simulink model "MPC_TRAJ"  (R2025b)
settings: Solver=VariableStepAuto  StartTime=0.0  StopTime=10  RelTol=1e-3
InitFcn:
  | clear; clc; close all;
  | 
  | % System parameters
  | m = 0.2;
  | M = 1;
  | g = 9.81;
  | bc = 0.1;
  | bp = 0.05;
  | l0 = 0.5;
  | theta0 = 0;
  | x0 = -0.5; % or -5
  | 
  | % NMPC horizons and constraints
  | Ts = 0.05;
  | prediction_horizon = 25;
  | control_horizon = 5;
  | 
  | theta_max = deg2rad(15);
  | theta_min = -theta_max;
  | l_max = 1.5; l_min = 0.1;
  | f_max = 50; f_min = -f_max;
  | l_ddot_max = 5; l_ddot_min = -l_ddot_max;
  | 
  | % NMPC object configuration
  | nx = 6; % States: [x, x_dot, theta, theta_dot, l, l_dot]
  | ny = 6; % Outputs
  | nu = 2; % Inputs: [F, l_ddot]
  | 
  | nlobj = nlmpc(nx, ny, nu);
  | nlobj.Model.StateFcn = "CraneStateFcn";
  | nlobj.Ts = Ts;
  | nlobj.PredictionHorizon = prediction_horizon;
  | nlobj.ControlHorizon = control_horizon;
  | 
  | % Set HARD state constraints
  | nlobj.States(3).Min = theta_min; nlobj.States(3).Max = theta_max;
  | nlobj.States(5).Min = l_min; nlobj.States(5).Max = l_max;
  | 
  | % Set MV hard constraints
  | nlobj.MV(1).Min = f_min; nlobj.MV(1).Max = f_max;
  | nlobj.MV(2).Min = l_ddot_min; nlobj.MV(2).Max = l_ddot_max;
  | 
  | % Distance-Invariant Tuning Weights
  | % OutputVariables: [x, x_dot, theta, theta_dot, l, l_dot]
  | % x weight reduced to allow tracking flexibility without constraint violation
  | nlobj.Weights.OutputVariables = [150, 20, 300, 20, 50, 10];
  | 
  | % ManipulatedVariables: [F, l_ddot]
  | nlobj.Weights.ManipulatedVariables = [1, 1];
  | 
  | % ManipulatedVariablesRate: [F_rate, l_ddot_rate]
  | % Heavily penalized to enforce smooth control actions, preventing hard constraint hits
  | nlobj.Weights.ManipulatedVariablesRate = [150, 150];
  | 
  | % Optimization solver settings
  | nlobj.Optimization.SolverOptions.Algorithm = 'sqp';
  | nlobj.Optimization.SolverOptions.MaxIterations = 200;
  | % Increase tolerance slightly to help the solver in tight constraint scenarios
  | nlobj.Optimization.SolverOptions.StepTolerance = 1e-4;
  | 
  | % Trajectory and feedforward parameters
  | v_max = 1.0;
  | a_max = 2.0;
  | traj_params = [x0, v_max, a_max, M, m, bc, l0];
model workspace (MAT data in the model file):
  Sig = Simulink.Signal
  Sig.Dimensions = -1
  Sig.DimensionsMode = 'auto'
  Sig.Complexity = 'auto'
  Sig.SampleTime = -1
  Sig.SamplingMode = 'auto'
  Sig.DataType = 'auto'
values from neighbouring files (symbols this model uses):
  L = x_target - x0    [TrajectoryGenerator.m]
  s = 10 * tau ^ 3 - 15 * tau ^ 4 + 6 * tau ^ 5    [TrajectoryGenerator.m]
undefined symbols (not defined in the file or in its folder): X, Y, Z
libraries: sm_lib x13, nesl_utility x7, mpclib x1
settings Model: Creator=JNemune  LastModifiedBy=JNemune

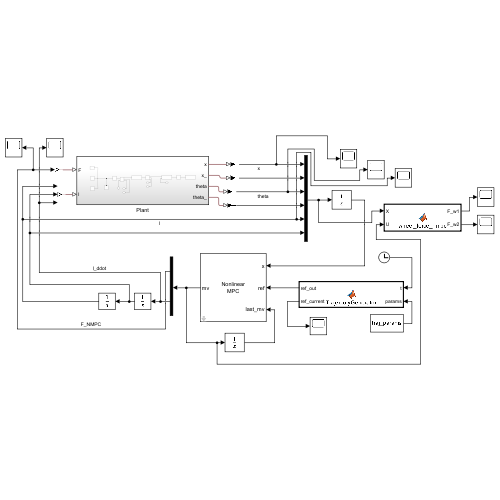
[thumbnail: Simulink's stored preview of the top-level diagram]
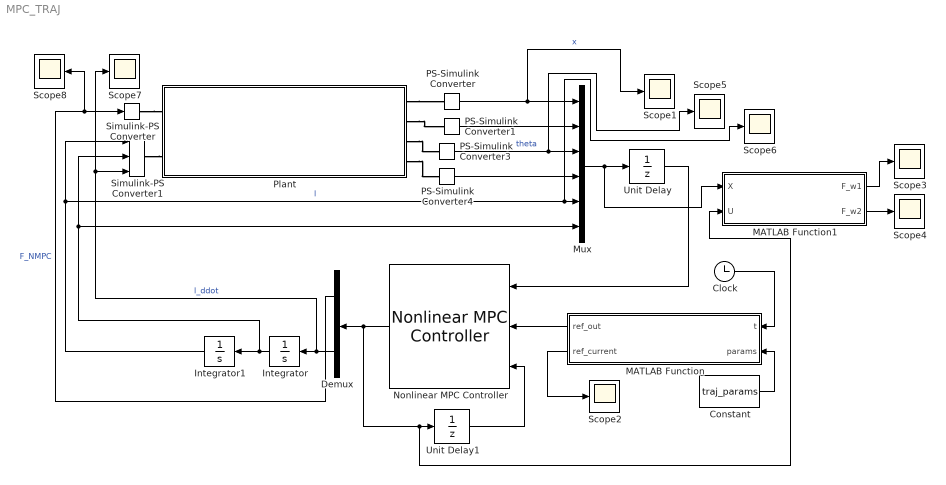
== system MPC_TRAJ ==
  Clock : Clock
  Constant : Constant  Value=traj_params
  Demux : Demux  Outputs=2
  Integrator : Integrator
  Integrator1 : Integrator  InitialCondition=l0
  MATLAB Function : MATLAB Function  TreatAsAtomicUnit=on
  MATLAB Function1 : MATLAB Function  TreatAsAtomicUnit=on
  Mux : Mux  Inputs=6
  Nonlinear MPC Controller : mpclib/Nonlinear MPC Controller  nlmpcobj=nlobj  UseObjectTs=on  UseMEX=off  md_enabled=off  mvtarget_enabled=off  param_enabled=off  cost_enabled=off  mvseq_enabled=off  stateseq_enabled=off  ovseq_enabled=off  slack_enabled=off  status_enabled=off  ov_min=off  ov_max=off  mv_min=off  mv_max=off  mvrate_min=off  mvrate_max=off  state_min=off  state_max=off  ov_weight=off  mv_weight=off  mvrate_weight=off  ecr_weight=off  nlp_initialize=off
  PS-Simulink Converter{,1,3..4} (4 alike) : nesl_utility/PS-Simulink Converter  PhysicalDomain=network_engine_domain  SubClassName=ps_output  LeftPortType=input  RightPortType=output  PseudoPeriodic=off  Frequencies=[]  VectorFormat=inherit  Unit=inherit  AffineConversion=off
  Plant : Subsystem
  Scope{1..8} (8 alike) : Scope
      Scope1 settings: Title=Plant Input (F, l_ddot)  ActiveDisplayYMinimum=-0.57069229240965214  ActiveDisplayYMaximum=0.1182567265577066
      Scope2 settings: ActiveDisplayYMinimum=-0.5625  ActiveDisplayYMaximum=0.062499999999999986  DataLoggingVariableName=ScopeData2
      Scope3 settings: Title=Plant Input (F, l_ddot)  ActiveDisplayYMinimum=5.8532583517724026  ActiveDisplayYMaximum=5.9075728848445683  DataLoggingVariableName=ScopeData3
      Scope4 settings: Title=Plant Input (F, l_ddot)  ActiveDisplayYMinimum=5.8611422440219316  ActiveDisplayYMaximum=5.9241092198238494  DataLoggingVariableName=ScopeData4
      Scope5 settings: Title=Plant Input (F, l_ddot)  ActiveDisplayYMinimum=-0.093511798344871486  ActiveDisplayYMaximum=0.060809549458767209
      Scope6 settings: Title=Plant Input (F, l_ddot)  ActiveDisplayYMinimum=0.49743738451947506  ActiveDisplayYMaximum=0.510974024582042  DataLoggingVariableName=ScopeData5
      Scope7 settings: Title=Plant Input (F, l_ddot)  ActiveDisplayYMinimum=-0.039593269711448255  ActiveDisplayYMaximum=0.049854556653327248  DataLoggingVariableName=ScopeData6
      Scope8 settings: Title=Plant Input (F, l_ddot)  ActiveDisplayYMinimum=-0.62140528534348749  ActiveDisplayYMaximum=0.7248047355020627  DataLoggingVariableName=ScopeData7
  Simulink-PS Converter : nesl_utility/Simulink-PS Converter  PhysicalDomain=network_engine_domain  SubClassName=ps_input  LeftPortType=input  RightPortType=output  PseudoPeriodic=off  Frequencies=[]  NoiseDistribution=none  NoiseParameters=[]  Unit=1  AffineConversion=off  FilteringAndDerivatives=provide  SimscapeFilterOrder=1  InputFilterTimeConstant=0.001  UdotUserProvided=0
  Simulink-PS Converter1 : nesl_utility/Simulink-PS Converter  PhysicalDomain=network_engine_domain  SubClassName=ps_input  LeftPortType=input  RightPortType=output  PseudoPeriodic=off  Frequencies=[]  NoiseDistribution=none  NoiseParameters=[]  Unit=1  AffineConversion=off  FilteringAndDerivatives=provide  SimscapeFilterOrder=1  InputFilterTimeConstant=0.001  UdotUserProvided=2
  Unit Delay : UnitDelay  InitialCondition=[0, 0, theta0, 0, l0, 0]  SampleTime=Ts  HasFrameUpgradeWarning=on
  Unit Delay1 : UnitDelay  InitialCondition=[0, 0]  SampleTime=Ts  HasFrameUpgradeWarning=on
  wires:
  PS-Simulink Converter1/1 -> Mux/2
  Integrator/1 -> Simulink-PS Converter1/2, Mux/6, Integrator1/1
  MATLAB Function/1(ref_out) -> Nonlinear MPC Controller/2
  Nonlinear MPC Controller/1 -> MATLAB Function1/2(U), Unit Delay1/1, Demux/1
  Integrator1/1 -> Simulink-PS Converter1/1, Scope6/1, Mux/5  "l"
  PS-Simulink Converter4/1 -> Mux/4
  Mux/1 -> MATLAB Function1/1(X), Unit Delay/1
  Unit Delay/1 -> Nonlinear MPC Controller/1
  Unit Delay1/1 -> Nonlinear MPC Controller/3
  PS-Simulink Converter3/1 -> Scope5/1, Mux/3  "theta"
  PS-Simulink Converter/1 -> Scope1/1, Mux/1  "x"
  Demux/2 -> Scope7/1, Simulink-PS Converter1/3, Integrator/1  "l_ddot"
  Demux/1 -> Scope8/1, Simulink-PS Converter/1  "F_NMPC"
  Clock/1 -> MATLAB Function/1(t)
  Constant/1 -> MATLAB Function/2(params)
  MATLAB Function/2(ref_current) -> Scope2/1
  MATLAB Function1/1(F_w1) -> Scope3/1
  MATLAB Function1/2(F_w2) -> Scope4/1
  connections:
  Plant/RConn2 -- PS-Simulink Converter1/LConn1
  Simulink-PS Converter1/RConn1 -- Plant/LConn2
  Simulink-PS Converter/RConn1 -- Plant/LConn1
  Plant/RConn3 -- PS-Simulink Converter3/LConn1
  Plant/RConn1 -- PS-Simulink Converter/LConn1
  Plant/RConn4 -- PS-Simulink Converter4/LConn1

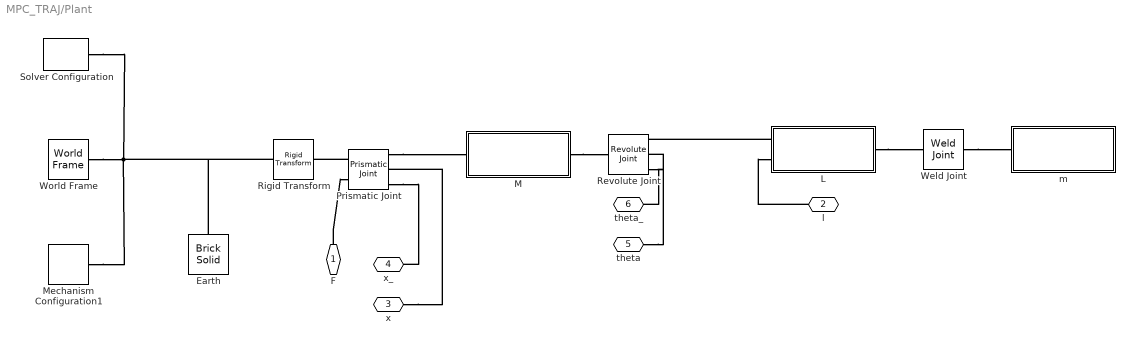
== system MPC_TRAJ/Plant ==
  Earth : sm_lib/Body Elements/Brick Solid  BrickDimensions=[1000 1 1]  BrickDimensionsUnits=mm  ExportEntireGeometry=off  InertiaType=CalculateFromGeometry  BasedOnType=Density  Density=1000  DensityUnits=kg/m^3  Mass=1  MassUnits=kg  CenterOfMass=[0 0 0]  CenterOfMassUnits=m  MomentsOfInertia=[1 1 1]  MomentsOfInertiaUnits=kg*m^2  ProductsOfInertia=[0 0 0]  ProductsOfInertiaUnits=kg*m^2  GraphicType=FromGeometry  MarkerShape=Sphere  MarkerSize=10  GraphicVisPropType=SimpleVisualProperties  GraphicDiffuseColor=[0.5 0.5 0.5]  GraphicOpacity=1.0  GraphicSpecularColor=[0.5 0.5 0.5 1.0]  GraphicAmbientColor=[0.15 0.15 0.15 1.0]  GraphicEmissiveColor=[0.0 0.0 0.0 1.0]  GraphicShininess=75  DoExposeReferenceFrame=on  SerializedFrames=<Frames/>
  L : Subsystem
  M : Subsystem
  Mechanism Configuration1 : sm_lib/Utilities/Mechanism Configuration  UniformGravity=Constant  GravityVector=[0 0 -g]  GravityVectorUnits=m/s^2  LinearizationDelta=0.001  JointModeTransitionNonlinearIterations=2
  Prismatic Joint : sm_lib/Joints/Prismatic Joint  JointMode=Normal  CompositeWrenchDir=FollowerOnBase  CompositeWrenchFrame=BaseFrame  SenseConstraintForce=off  SenseConstraintTorque=off  SenseTotalForce=off  SenseTotalTorque=off  PositionTargetSpecify=on  PositionTargetPriority=High  PositionTargetValue=x0  PositionTargetValueUnits=m  VelocityTargetSpecify=off  VelocityTargetPriority=High  VelocityTargetValue=0  VelocityTargetValueUnits=m/s  EquilibriumPosition=0  EquilibriumPositionUnits=m  SpringStiffness=0  SpringStiffnessUnits=N/m  DampingCoefficient=bc  DampingCoefficientUnits=N/(m/s)  LowerLimitSpecify=off  LowerLimitBound=-1  LowerLimitBoundUnits=m  LowerLimitStiffness=1e6  LowerLimitStiffnessUnits=N/m  LowerLimitDamping=1e3  LowerLimitDampingUnits=N/(m/s)  LowerLimitTransitionRegionWidth=1e-4  LowerLimitTransitionRegionWidthUnits=m  UpperLimitSpecify=off  UpperLimitBound=1  UpperLimitBoundUnits=m  UpperLimitStiffness=1e6  UpperLimitStiffnessUnits=N/m  UpperLimitDamping=1e3  UpperLimitDampingUnits=N/(m/s)  UpperLimitTransitionRegionWidth=1e-4  UpperLimitTransitionRegionWidthUnits=m  TorqueActuationMode=InputTorque  MotionActuationMode=ComputedMotion  SensePosition=on  SenseVelocity=on  SenseAcceleration=off  SenseTorqueForce=off  SenseLowerLimitTorqueForce=off  SenseUpperLimitTorqueForce=off
  Revolute Joint : sm_lib/Joints/Revolute Joint  JointMode=Normal  CompositeWrenchDir=FollowerOnBase  CompositeWrenchFrame=BaseFrame  SenseConstraintForce=off  SenseConstraintTorque=off  SenseTotalForce=off  SenseTotalTorque=off  PositionTargetSpecify=on  PositionTargetPriority=High  PositionTargetValue=theta0  PositionTargetValueUnits=rad  VelocityTargetSpecify=off  VelocityTargetPriority=High  VelocityTargetValue=0  VelocityTargetValueUnits=deg/s  EquilibriumPosition=0  EquilibriumPositionUnits=deg  SpringStiffness=0  SpringStiffnessUnits=N*m/deg  DampingCoefficient=bp  DampingCoefficientUnits=N*m*s/rad  LowerLimitSpecify=off  LowerLimitBound=-90  LowerLimitBoundUnits=deg  LowerLimitStiffness=1e4  LowerLimitStiffnessUnits=N*m/deg  LowerLimitDamping=10  LowerLimitDampingUnits=N*m/(deg/s)  LowerLimitTransitionRegionWidth=0.1  LowerLimitTransitionRegionWidthUnits=deg  UpperLimitSpecify=off  UpperLimitBound=90  UpperLimitBoundUnits=deg  UpperLimitStiffness=1e4  UpperLimitStiffnessUnits=N*m/deg  UpperLimitDamping=10  UpperLimitDampingUnits=N*m/(deg/s)  UpperLimitTransitionRegionWidth=0.1  UpperLimitTransitionRegionWidthUnits=deg  TorqueActuationMode=NoTorque  MotionActuationMode=ComputedMotion  SensePosition=on  SenseVelocity=on  SenseAcceleration=off  SenseTorqueForce=off  SenseLowerLimitTorqueForce=off  SenseUpperLimitTorqueForce=off
  Rigid Transform : sm_lib/Frames and Transforms/Rigid Transform  RotationMethod=StandardAxis  FollAlignAxisA=+X  BaseAlignAxisA=+Y  FollAlignAxisB=+Y  BaseAlignAxisB=+Z  RotationStandardAxis=+Y  RotationAngle=90  RotationAngleUnits=deg  RotationArbitraryAxis=[0 0 1]  RotationSequenceAxes=FollowerAxes  RotationSequence=XYX  RotationSequenceAngles=[0 0 0]  RotationSequenceAnglesUnits=deg  RotationMatrix=[1 0 0; 0 1 0; 0 0 1]  Quaternion=[1 0 0 0]  TranslationMethod=None  TranslationCartesianOffset=[x0 0 0]  TranslationCartesianOffsetUnits=m  TranslationStandardAxis=+Z  TranslationStandardOffset=0  TranslationStandardOffsetUnits=m  TranslationROffset=0  TranslationROffsetUnits=m  TranslationThetaOffset=0  TranslationThetaOffsetUnits=deg  TranslationZOffset=0  TranslationZOffsetUnits=m
  Solver Configuration : nesl_utility/Solver Configuration  PhysicalDomain=network_engine_domain  SubClassName=solver  LeftPortType=input  RightPortType=generic  Tones=[]  Harmonics=[]  SimulateNoise=off  Profile=off  UseLocalSampling=off  EnableSwitchedLinearOptims=on  FrequencyDomain=off  UseCCode=off  RelTol=0.001  AbsTol=0.001  MinStep=1e-09  ToWorkspace=off  RevertToSquareIcSolve=off  NumHomotopyIterations=100  PhasorMode=off  PhasorModeNumHarmonics=1  ConsistencySolver=NEWTON_XTOL_AFTER_FTOL  IndexReductionMethod=DerivativeReplacement  DoDC=off  ResidualTolerance=1e-09  ConsistencyTolSource=GLOBAL  ConsistencyAbsTol=0.001  ConsistencyRelTol=0.001  ConsistencyTolFactor=0.001  UseLocalSolver=off  LocalSolverChoice=NE_BACKWARD_EULER_ADVANCER  ResolveIndetEquations=on  FunctionEvalNumThread=1  LocalSolverSampleTime=0.001  DoFixedCost=off  MaxNonlinIter=3  MaxModeIter=2  ComputeImpulses=off  ImpulseIterations=2  LinearAlgebra=auto  LinearAlgebraNumThread=0  EquationFormulation=NE_TIME_EF  DelaysMemoryBudget=1024  AutomaticFiltering=on  FilteringTimeConstant=0.001  PartitionStorageMethod=AS_NEEDED  PartitionMemoryBudget=1024  PartitionMethod=ROBUST  MultibodyUseLocalSolver=off  MultibodyLocalSolverChoice=ODE1  MultibodyLocalSolverSampleTime=0.001
  Weld Joint : sm_lib/Joints/Weld Joint  JointMode=Normal  CompositeWrenchDir=FollowerOnBase  CompositeWrenchFrame=BaseFrame  SenseConstraintForce=off  SenseConstraintTorque=off  SenseTotalForce=off  SenseTotalTorque=off
  World Frame : sm_lib/Frames and Transforms/World Frame
  m : Subsystem
  F : PMIOPort  Side=Left
  l : PMIOPort  Port=2  Side=Left
  x : PMIOPort  Port=3  Side=Right
  x_ : PMIOPort  Port=4  Side=Right
  theta : PMIOPort  Port=5  Side=Right
  theta_ : PMIOPort  Port=6  Side=Right
  connections:
  Solver Configuration/RConn1 -- Earth/RConn1 -- Rigid Transform/LConn1 -- World Frame/RConn1 -- Mechanism Configuration1/RConn1
  Prismatic Joint/LConn1 -- Rigid Transform/RConn1
  Weld Joint/RConn1 -- m/LConn1
  L/LConn1 -- Revolute Joint/RConn1
  M/RConn1 -- Revolute Joint/LConn1
  L/RConn1 -- Weld Joint/LConn1
  Prismatic Joint/RConn1 -- M/LConn1
  l/RConn1 -- L/LConn2
  F/RConn1 -- Prismatic Joint/LConn2
  Revolute Joint/RConn3 -- theta_/RConn1
  Prismatic Joint/RConn3 -- x_/RConn1
  x/RConn1 -- Prismatic Joint/RConn2
  theta/RConn1 -- Revolute Joint/RConn2

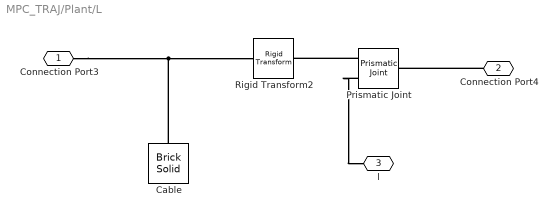
== system MPC_TRAJ/Plant/L ==
  Cable : sm_lib/Body Elements/Brick Solid  BrickDimensions=[l0, 0.001, 0.001]  BrickDimensionsUnits=m  ExportEntireGeometry=off  InertiaType=Custom  BasedOnType=Density  Density=1000  DensityUnits=kg/m^3  Mass=0  MassUnits=kg  CenterOfMass=[0 0 0]  CenterOfMassUnits=m  MomentsOfInertia=[0 0 0]  MomentsOfInertiaUnits=kg*m^2  ProductsOfInertia=[0 0 0]  ProductsOfInertiaUnits=kg*m^2  GraphicType=FromGeometry  MarkerShape=Frame  MarkerSize=10  GraphicVisPropType=SimpleVisualProperties  GraphicDiffuseColor=[0.5 0.5 0.5]  GraphicOpacity=1.0  GraphicSpecularColor=[0.5 0.5 0.5 1.0]  GraphicAmbientColor=[0.15 0.15 0.15 1.0]  GraphicEmissiveColor=[0.0 0.0 0.0 1.0]  GraphicShininess=75  DoExposeReferenceFrame=off  SerializedFrames=|
      | <Frames>
      | 
      |   <Frame>
      |     <Id>Frame1</Id>
      |     <Value>
      |       <Name>cable joint</Name>
      |       <Origin>
      |         <Source>GeometricFeature</Source>
      |         <FeatureName>-x -y +z point</FeatureName>
      |       </Origin>
      |       <PrimaryAxis>
      |         <DefinedDirection>+Z</DefinedDirection>
      |         <Source>ReferenceFrame</Source>
      |         <SourceDirection>+Z</SourceDirection>
      |         <FeatureName></FeatureName>
      |       </PrimaryAxis>
      |       <SecondaryAxis>
      |         <DefinedDirection>+X</DefinedDirection>
      |         <Source>ReferenceFrame</Source>
      |         <SourceDirection>+X</SourceDirection>
      |         <FeatureName></FeatureName>
      |       </SecondaryAxis>
      |     </Value>
      |   </Frame>
      | 
      | </Frames>
  Prismatic Joint : sm_lib/Joints/Prismatic Joint  JointMode=Normal  CompositeWrenchDir=FollowerOnBase  CompositeWrenchFrame=BaseFrame  SenseConstraintForce=off  SenseConstraintTorque=off  SenseTotalForce=off  SenseTotalTorque=off  PositionTargetSpecify=off  PositionTargetPriority=High  PositionTargetValue=l0  PositionTargetValueUnits=m  VelocityTargetSpecify=off  VelocityTargetPriority=High  VelocityTargetValue=0  VelocityTargetValueUnits=m/s  EquilibriumPosition=0  EquilibriumPositionUnits=m  SpringStiffness=0  SpringStiffnessUnits=N/m  DampingCoefficient=0  DampingCoefficientUnits=N/(m/s)  LowerLimitSpecify=off  LowerLimitBound=-1  LowerLimitBoundUnits=m  LowerLimitStiffness=1e6  LowerLimitStiffnessUnits=N/m  LowerLimitDamping=1e3  LowerLimitDampingUnits=N/(m/s)  LowerLimitTransitionRegionWidth=1e-4  LowerLimitTransitionRegionWidthUnits=m  UpperLimitSpecify=off  UpperLimitBound=1  UpperLimitBoundUnits=m  UpperLimitStiffness=1e6  UpperLimitStiffnessUnits=N/m  UpperLimitDamping=1e3  UpperLimitDampingUnits=N/(m/s)  UpperLimitTransitionRegionWidth=1e-4  UpperLimitTransitionRegionWidthUnits=m  TorqueActuationMode=ComputedTorque  MotionActuationMode=InputMotion  SensePosition=off  SenseVelocity=off  SenseAcceleration=off  SenseTorqueForce=off  SenseLowerLimitTorqueForce=off  SenseUpperLimitTorqueForce=off
  Rigid Transform2 : sm_lib/Frames and Transforms/Rigid Transform  RotationMethod=StandardAxis  FollAlignAxisA=+X  BaseAlignAxisA=+Y  FollAlignAxisB=+Y  BaseAlignAxisB=+Z  RotationStandardAxis=+Y  RotationAngle=pi/2  RotationAngleUnits=rad  RotationArbitraryAxis=[0 0 1]  RotationSequenceAxes=FollowerAxes  RotationSequence=XYX  RotationSequenceAngles=[0 0 0]  RotationSequenceAnglesUnits=deg  RotationMatrix=[1 0 0; 0 1 0; 0 0 1]  Quaternion=[1 0 0 0]  TranslationMethod=None  TranslationCartesianOffset=[L/2*cos(theta0), L/2*sin(theta0), 0]  TranslationCartesianOffsetUnits=m  TranslationStandardAxis=+Z  TranslationStandardOffset=0  TranslationStandardOffsetUnits=m  TranslationROffset=0  TranslationROffsetUnits=m  TranslationThetaOffset=0  TranslationThetaOffsetUnits=deg  TranslationZOffset=0  TranslationZOffsetUnits=m
  Connection Port3 : PMIOPort  Side=Left
  Connection Port4 : PMIOPort  Port=2  Side=Right
  l : PMIOPort  Port=3  Side=Left
  connections:
  Prismatic Joint/LConn1 -- Rigid Transform2/RConn1
  Connection Port3/RConn1 -- Cable/LConn1 -- Rigid Transform2/LConn1
  Connection Port4/RConn1 -- Prismatic Joint/RConn1
  Prismatic Joint/LConn2 -- l/RConn1

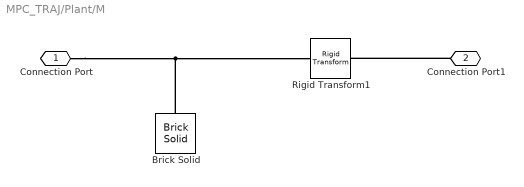
== system MPC_TRAJ/Plant/M ==
  Brick Solid : sm_lib/Body Elements/Brick Solid  BrickDimensions=[1 1 1]  BrickDimensionsUnits=mm  ExportEntireGeometry=off  InertiaType=PointMass  BasedOnType=Density  Density=1000  DensityUnits=kg/m^3  Mass=M  MassUnits=kg  CenterOfMass=[0 0 0]  CenterOfMassUnits=m  MomentsOfInertia=[1 1 1]  MomentsOfInertiaUnits=kg*m^2  ProductsOfInertia=[0 0 0]  ProductsOfInertiaUnits=kg*m^2  GraphicType=FromGeometry  MarkerShape=Sphere  MarkerSize=10  GraphicVisPropType=SimpleVisualProperties  GraphicDiffuseColor=[0.5 0.5 0.5]  GraphicOpacity=1.0  GraphicSpecularColor=[0.5 0.5 0.5 1.0]  GraphicAmbientColor=[0.15 0.15 0.15 1.0]  GraphicEmissiveColor=[0.0 0.0 0.0 1.0]  GraphicShininess=75  DoExposeReferenceFrame=on  SerializedFrames=<Frames/>
  Rigid Transform1 : sm_lib/Frames and Transforms/Rigid Transform  RotationMethod=StandardAxis  FollAlignAxisA=+X  BaseAlignAxisA=+Y  FollAlignAxisB=+Y  BaseAlignAxisB=+Z  RotationStandardAxis=+X  RotationAngle=90  RotationAngleUnits=deg  RotationArbitraryAxis=[0 0 1]  RotationSequenceAxes=FollowerAxes  RotationSequence=XYX  RotationSequenceAngles=[0 0 0]  RotationSequenceAnglesUnits=deg  RotationMatrix=[1 0 0; 0 1 0; 0 0 1]  Quaternion=[1 0 0 0]  TranslationMethod=None  TranslationCartesianOffset=[0 0 0]  TranslationCartesianOffsetUnits=m  TranslationStandardAxis=+Z  TranslationStandardOffset=0  TranslationStandardOffsetUnits=m  TranslationROffset=0  TranslationROffsetUnits=m  TranslationThetaOffset=0  TranslationThetaOffsetUnits=deg  TranslationZOffset=0  TranslationZOffsetUnits=m
  Connection Port : PMIOPort  Side=Left
  Connection Port1 : PMIOPort  Port=2  Side=Right
  connections:
  Brick Solid/RConn1 -- Connection Port/RConn1 -- Rigid Transform1/LConn1
  Connection Port1/RConn1 -- Rigid Transform1/RConn1

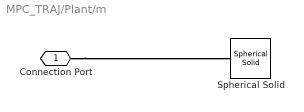
== system MPC_TRAJ/Plant/m ==
  Spherical Solid : sm_lib/Body Elements/Spherical Solid  SphereRadius=1  SphereRadiusUnits=cm  ExportEntireGeometry=off  InertiaType=PointMass  BasedOnType=Density  Density=1000  DensityUnits=kg/m^3  Mass=m  MassUnits=kg  CenterOfMass=[0 0 0]  CenterOfMassUnits=m  MomentsOfInertia=[1 1 1]  MomentsOfInertiaUnits=kg*m^2  ProductsOfInertia=[0 0 0]  ProductsOfInertiaUnits=kg*m^2  GraphicType=FromGeometry  MarkerShape=Sphere  MarkerSize=10  GraphicVisPropType=SimpleVisualProperties  GraphicDiffuseColor=[0.5 0.5 0.5]  GraphicOpacity=1.0  GraphicSpecularColor=[0.5 0.5 0.5 1.0]  GraphicAmbientColor=[0.15 0.15 0.15 1.0]  GraphicEmissiveColor=[0.0 0.0 0.0 1.0]  GraphicShininess=75  DoExposeReferenceFrame=on  SerializedFrames=<Frames/>
  Connection Port : PMIOPort  Side=Left
  connections:
  Connection Port/RConn1 -- Spherical Solid/RConn1

== matlab function MPC_TRAJ/MATLAB Function1 ==
  data: X input; F_w1 output; U input; F_w2 output
function [F_w1, F_w2] = wheel_force_nmpc(X, U)
    % Extract states for NMPC architecture
    x_dot = X(2);
    theta = X(3);
    theta_dot = X(4);
    l = X(5);
    l_dot = X(6);

    % Prevent singularity at l = 0
    if l < 0.01
        l = 0.01;
    end

    % Extract inputs
    F = U(1);
    l_ddot = U(2);

    % System physical parameters
    m = 0.2;
    M = 1.0;
    g = 9.81;
    bc = 0.1;
    bp = 0.05;
    D1 = 0.2;
    D2 = 0.1;

    % Precompute trigonometric terms
    s = sin(theta);
    c = cos(theta);

    % Calculate theta_ddot using analytical inversion
    RHS1 = F - bc * x_dot - m * l_ddot * s ...
        - 2 * m * l_dot * theta_dot * c ...
        + m * l * theta_dot ^ 2 * s;

    RHS2 = -2 * m * l * l_dot * theta_dot ...
        - m * g * l * s ...
        - bp * theta_dot;

    theta_ddot = ((M + m) * RHS2 - m * l * c * RHS1) / (m * l ^ 2 * (M + m * s ^ 2));

    % Payload vertical acceleration via local polar coordinates
    a_radial = l_ddot - l * theta_dot ^ 2;
    a_tang = l * theta_ddot + 2 * l_dot * theta_dot;
    y_p_ddot = -a_radial * c + a_tang * s;

    % Wheel load calculations
    F_sum = (M + m) * g + m * y_p_ddot;
    F_diff = (D2 * bc * x_dot - bp * theta_dot) / D1;

    % Final vertical loads on left and right wheel sets
    F_w1 = (F_sum - F_diff) / 2;
    F_w2 = (F_sum + F_diff) / 2;
end

== matlab function MPC_TRAJ/MATLAB Function ==
  data: t input; ref_out output; params input; ref_current output
function [ref_out, ref_current] = TrajectoryGenerator(t, params)
    % Extract parameters
    x0 = params(1); v_max = params(2); a_max = params(3);
    l0 = params(7);

    x_target = 0.0;
    L = x_target - x0;
    D = abs(L);

    % NMPC settings
    Np = 25;
    Ts = 0.05;

    % Initialize reference matrix (Np x 6)
    ref_out = zeros(Np, 6);

    % Handle zero displacement
    if D < 1e-4
        ref_out = repmat([x_target, 0, 0, 0, l0, 0], Np, 1);
        ref_current = ref_out(1, :);
        return;
    end

    % Calculate minimum travel time constraints
    T_v = (15/8) * (D / v_max);
    T_a = sqrt((5.77 * D) / a_max);
    T_p = 2 * pi * sqrt(l0 / 9.81);

    % Select maximum required time for safety and sway suppression
    T = max([T_v, T_a, 1.5 * T_p]);

    % Generate future references over the prediction horizon
    for k = 1:Np
        t_future = t + (k - 1) * Ts;
        tau = max(0.0, min(t_future / T, 1.0));

        % 5th-order S-curve polynomial
        s = 10 * tau ^ 3 - 15 * tau ^ 4 + 6 * tau ^ 5;
        s_dot = (30 * tau ^ 2 - 60 * tau ^ 3 + 30 * tau ^ 4) / T;

        % Set reference state: [x, x_dot, theta, theta_dot, l, l_dot]
        % Target sway angle is strictly zero
        ref_out(k, :) = [x0 + L * s, L * s_dot, 0, 0, l0, 0];
    end

    % Extract current reference for feedback calculations
    ref_current = ref_out(1, :);
end
